simulink model "servo_lqr"  (R2015a)
settings: Solver=ode45  StartTime=0.0  StopTime=10.0  RelTol=1e-3
values from neighbouring files (symbols this model uses):
  A = [0 1 ... (first row only)    [optimal_care.m]    (also in optimal_hamilton.m; optimal_servo.m = [ 0 1 0 0)
  B = [0 1]'    [optimal_care.m]    (also in optimal_hamilton.m; optimal_servo.m = [0 2 0 0]')
  C = [ 0 0 1 0]    [optimal_servo.m]
  Fa = [-K+2*G*inv(P22)*P12' 1]*inv(M0)*[zeros(4,1);1]    [optimal_servo.m]
  Fb = -2*G*inv(P22)*P12'    [optimal_servo.m]
  G = -inv(Re)*B'*P12    [optimal_servo.m]
  K = -inv(R)*B'*P    [optimal_care.m]    (also in optimal_hamilton.m = -acker(A,B,lambda); optimal_servo.m = -inv(Re)*B'*P11)
  x0 = [1 0]'    [optimal_care.m]    (also in optimal_hamilton.m; optimal_servo.m = [0 0 0.25 0]')
settings Model: Creator=shohei  LastModifiedBy=shohei

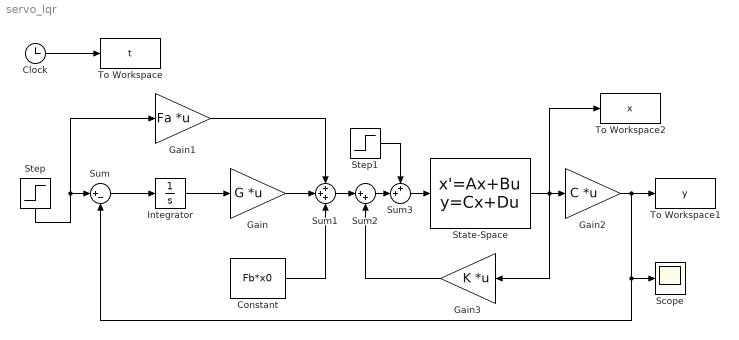
== system servo_lqr ==
  Clock : Clock
  Constant : Constant  Value=Fb*x0
  Gain : Gain  Gain=G  Multiplication=Matrix(K*u)
  Gain1 : Gain  Gain=Fa  Multiplication=Matrix(K*u)
  Gain2 : Gain  Gain=C  Multiplication=Matrix(K*u)
  Gain3 : Gain  Gain=K  Multiplication=Matrix(K*u)
  Integrator : Integrator
  Scope : Scope
  State-Space : StateSpace  A=A  B=B  C=eye(4)  D=zeros(4,1)  X0=x0
  Step : Step  Time=0  SampleTime=0
  Step1 : Step  Time=5  SampleTime=0
  Sum : Sum  Inputs=|+-
  Sum1 : Sum  Inputs=+++
  Sum2 : Sum  Inputs=|++
  Sum3 : Sum  Inputs=++|
  To Workspace : ToWorkspace  VariableName=t  SampleTime=-1
  To Workspace1 : ToWorkspace  VariableName=y  SampleTime=-1
  To Workspace2 : ToWorkspace  VariableName=x  SampleTime=-1
  wires:
  Clock/1 -> To Workspace/1
  Step/1 -> Gain1/1, Sum/1
  Sum/1 -> Integrator/1
  Integrator/1 -> Gain/1
  Gain/1 -> Sum1/2
  Gain1/1 -> Sum1/1
  Constant/1 -> Sum1/3
  Sum3/1 -> State-Space/1
  Step1/1 -> Sum3/1
  State-Space/1 -> To Workspace2/1, Gain3/1, Gain2/1
  Gain2/1 -> Sum/2, Scope/1, To Workspace1/1
  Sum1/1 -> Sum2/1
  Sum2/1 -> Sum3/2
  Gain3/1 -> Sum2/2
